simulink subsystem "charge_trasfer_controller"  (R2023b)
settings: Solver=VariableStepAuto  StartTime=0.0  StopTime=10.0  RelTol=1e-3
settings Model: Creator=10661025  LastModifiedBy=10661025

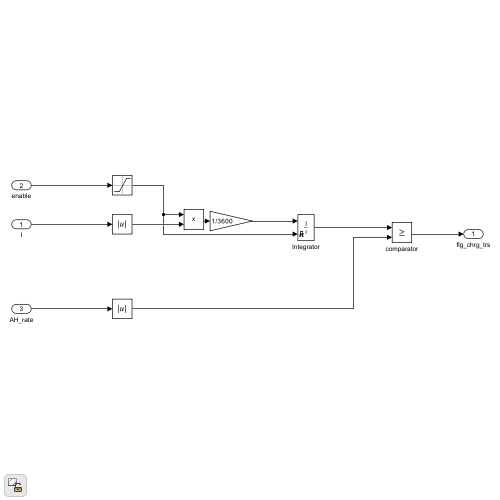
[thumbnail: Simulink's stored preview of the top-level diagram]
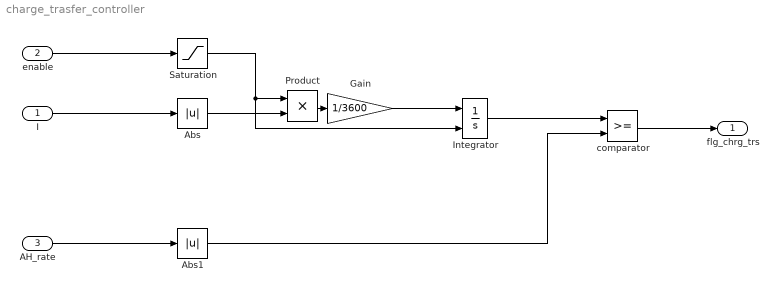
== system charge_trasfer_controller ==
  I : Inport
  enable : Inport  Port=2
  AH_rate : Inport  Port=3
  Abs : Abs  SaturateOnIntegerOverflow=off
  Abs1 : Abs  SaturateOnIntegerOverflow=off
  Gain : Gain  Gain=1/3600
  Integrator : Integrator  ExternalReset=either
  Product : Product
  Saturation : Saturate  UpperLimit=1  LowerLimit=0
  comparator : RelationalOperator  OutDataTypeStr=boolean  RndMeth=Simplest  InputSameDT=off
  flg_chrg_trs : Outport
  wires:
  comparator/1 -> flg_chrg_trs/1
  Saturation/1 -> Integrator/2, Product/1
  AH_rate/1 -> Abs1/1
  Abs/1 -> Product/2
  Integrator/1 -> comparator/1
  Product/1 -> Gain/1
  enable/1 -> Saturation/1
  Gain/1 -> Integrator/1
  I/1 -> Abs/1
  Abs1/1 -> comparator/2
